simulink model "problem1_old"  (Simulink 8.9)
settings: Solver=VariableStepAuto  StartTime=0.0  StopTime=10.0  RelTol=1e-3
values from neighbouring files (symbols this model uses):
  b = 10    [constants.m]    (also in problem1.m)
  eo = 0.0005    [constants.m]    (also in problem1.m)
  k = 10    [constants.m]    (also in problem1.m)
  m = 0.1    [constants.m]    (also in problem1.m)
  p = 0.000015    (= 1.5e-05)    [constants.m]    (also in problem1.m)
  z0 = 0.2    [constants.m]    (also in problem1.m)
settings Model: Creator=Janne  LastModifiedBy=Janne
settings DataIOCC: LimitDataPoints=off  SaveFormat=Dataset  SignalLoggingSaveFormat=Dataset
settings OptimizationCC: LifeSpan=auto
settings DebuggingCC: UnderspecifiedInitializationDetection=Simplified  MergeDetectMultiDrivingBlocksExec=error  FcnCallInpInsideContextMsg=error  StateNameClashWarn=none  SFUnexpectedBacktrackingDiag=error  SFNoUnconditionalDefaultTransitionDiag=error  SFExecutionAtInitializationDiag=warning
settings HardwareCC: ProdBitPerPointer=64  ProdBitPerSizeT=64  ProdBitPerPtrDiffT=64  ProdLargestAtomicFloat=Float  ProdIntDivRoundTo=Zero  ProdEndianess=LittleEndian  ProdWordSize=64  ProdHWDeviceType=Intel->x86-64 (Windows64)
settings ModelReferenceCC: PropagateSignalLabelsOutOfModel=on
settings SFSimCC: SimUseLocalCustomCode=on
settings RTWCC: RTWUseLocalCustomCode=on
settings GRTTargetCC: TargetLangStandard=C99 (ISO)  GeneratePreprocessorConditionals=Use local settings  CombineOutputUpdateFcns=on  GRTInterface=off
settings ConfigComp: CovMetricSettings=dwe  CovHtmlReporting=off  CovSaveCumulativeToWorkspaceVar=off  CovSaveSingleToWorkspaceVar=off  CovExternalEMLEnable=on

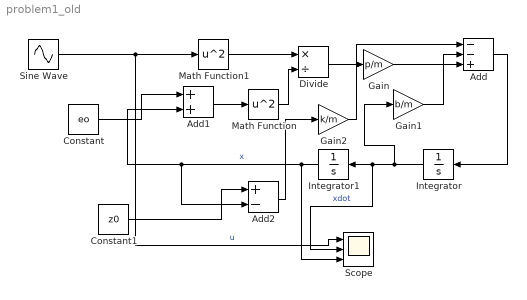
== system problem1_old ==
  Add : Sum  Inputs=--+
  Add1 : Sum
  Add2 : Sum  Inputs=+-
  Constant : Constant  Value=eo
  Constant1 : Constant  Value=z0
  Divide : Product  Inputs=*/
  Gain : Gain  Gain=p/m
  Gain1 : Gain  Gain=b/m
  Gain2 : Gain  Gain=k/m
  Integrator : Integrator
  Integrator1 : Integrator  InitialCondition=0.15
  Math Function : Math  Operator=square  SaturateOnIntegerOverflow=on
  Math Function1 : Math  Operator=square  SaturateOnIntegerOverflow=on
  Scope : Scope  NumInputPorts=3
  Sine Wave : Sin  Amplitude=10  Frequency=10  SampleTime=0
  wires:
  Add/1 -> Integrator/1
  Integrator/1 -> Gain1/1, Scope/2, Integrator1/1  "xdot"
  Integrator1/1 -> Scope/3, Add2/2, Add1/2  "x"
  Constant/1 -> Add1/1
  Add1/1 -> Math Function/1
  Sine Wave/1 -> Scope/1, Math Function1/1  "u"
  Math Function/1 -> Divide/2
  Math Function1/1 -> Divide/1
  Divide/1 -> Gain/1
  Gain/1 -> Add/3
  Add2/1 -> Gain2/1
  Gain1/1 -> Add/2
  Constant1/1 -> Add2/1
  Gain2/1 -> Add/1
